simulink model "EKG_Simulink"  (R2023b)
settings: Solver=VariableStepAuto  StartTime=0.0  StopTime=10.0  RelTol=1e-3
values from neighbouring files (symbols this model uses):
  C = 1    [EKG.m]
settings Model: Creator=mrado  LastModifiedBy=mrado

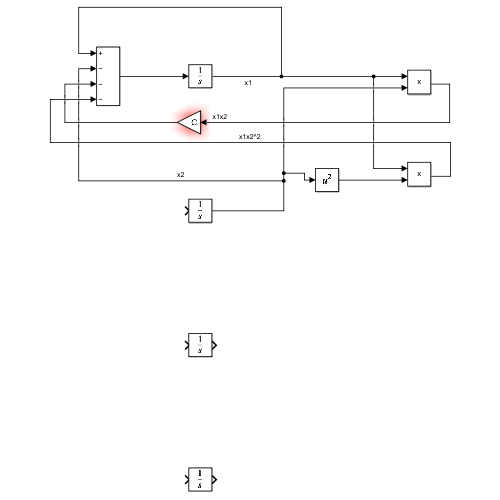
[thumbnail: Simulink's stored preview of the top-level diagram]
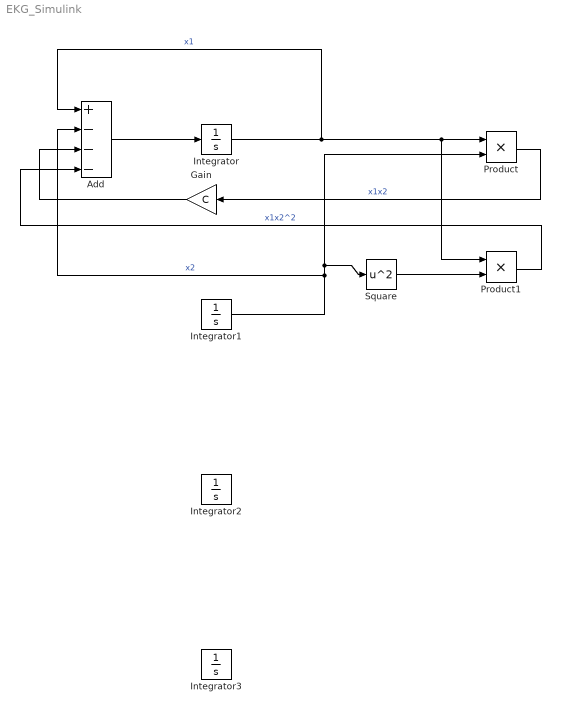
== system EKG_Simulink ==
  Add : Sum  Inputs=+---
  Gain : Gain  Gain=C
  Integrator{,1..3} (4 alike) : Integrator
  Product : Product
  Product1 : Product
  Square : Math  Operator=square
  wires:
  Add/1 -> Integrator/1
  Integrator/1 -> Product1/1, Product/1, Add/1  "x1"
  Integrator1/1 -> Square/1, Product/2, Add/2  "x2"
  Product/1 -> Gain/1  "x1x2"
  Square/1 -> Product1/2
  Product1/1 -> Add/4  "x1x2^2"
  Gain/1 -> Add/3
